simulink library "NeuroMuscularLibrary"  (R2014b)
settings: Solver=ode45  StartTime=0.0  StopTime=10.0  RelTol=1e-3
values from neighbouring files (symbols this model uses):
  c = 0.05    [BodyMechParams.m]
  c_jointstop = 0.3 / (pi/180)    (= 17.1887338539)    [BodyMechParams.m]
  DeltaThRef = 2e-3    (= 0.002)    [BodyMechParams.m]
  eref = 0.04    [BodyMechParams.m]
  footBallToAnkleDist = 0.16    [BodyMechParams.m]
  footBallToCenterDist = footLength/2    (= 0.1)    [BodyMechParams.m]
  footBallToHeelDist = footLength    (= 0.2)    [BodyMechParams.m]
  footCenterToCGDist = 0.14 - footBallToCenterDist    (= 0.04)    [BodyMechParams.m]
  footInertia = 0.005    [BodyMechParams.m]
  footLength = 0.2    [BodyMechParams.m]
  footMass = 1.25    [BodyMechParams.m]
  g = 9.80665    [BodyMechParams.m]
  groundTheta = [atan(diff(groundZ)./diff(groundX)), 0]    [generateGround.m]
  groundZ = groundZ * stepSize/(largestStep+eps)    [generateGround.m]
  hatHipToCenterDistLen = hatLength/2    (= 0.4)    [BodyMechParams.m]
  hatInertia = 3    [BodyMechParams.m]
  hatLeftHipToCenterDistWidth = .15    (= 0.15)    [BodyMechParams.m]
  hatLength = 0.8    [BodyMechParams.m]
  hatMass = 53.5    [BodyMechParams.m]
  hatThickness = 0.2    [BodyMechParams.m]
  hatWidth = 0.4    [BodyMechParams.m]
  K = 5    [BodyMechParams.m]
  k_gn = k_gz    (= 78453.2)    [BodyMechParams.m]
  k_gt = k_gz    (= 78453.2)    [BodyMechParams.m]
  k_pressure = hatMass * g / DeltaThRef    (= 262327.8875)    [BodyMechParams.m]
  loptGAS = 0.05    [BodyMechParams.m]
  loptGLU = 0.11    [BodyMechParams.m]
  loptHAM = 0.10    (= 0.1)    [BodyMechParams.m]
  loptHFL = 0.11    [BodyMechParams.m]
  loptSOL = 0.04    [BodyMechParams.m]
  loptTA = 0.06    [BodyMechParams.m]
  loptVAS = 0.08    [BodyMechParams.m]
  lslackGAS = 0.40    (= 0.4)    [BodyMechParams.m]
  lslackGLU = 0.13    [BodyMechParams.m]
  lslackHAM = 0.31    [BodyMechParams.m]
  lslackHFL = 0.10    (= 0.1)    [BodyMechParams.m]
  lslackSOL = 0.26    [BodyMechParams.m]
  lslackTA = 0.24    [BodyMechParams.m]
  lslackVAS = 0.23    [BodyMechParams.m]
  mu_slide = 0.8    [BodyMechParams.m]
  mu_stick = 0.9    [BodyMechParams.m]
  N = 1.5    [BodyMechParams.m]    (also in cmaes.m = size(x,1))
  phimaxGASa = 20*pi/180    (= 0.349065850399)    [BodyMechParams.m]
  phimaxGASk = 40*pi/180    (= 0.698131700798)    [BodyMechParams.m]
  phimaxHAMk = 0*pi/180    (= 0)    [BodyMechParams.m]
  phimaxSOL = 20*pi/180    (= 0.349065850399)    [BodyMechParams.m]
  phimaxTA = -10*pi/180    (= -0.174532925199)    [BodyMechParams.m]
  phimaxVAS = 15*pi/180    (= 0.261799387799)    [BodyMechParams.m]
  phirefGASa = -10*pi/180    (= -0.174532925199)    [BodyMechParams.m]
  phirefGASk = 15*pi/180    (= 0.261799387799)    [BodyMechParams.m]
  phirefGLU = -30*pi/180    (= -0.523598775598)    [BodyMechParams.m]
  phirefHAMh = -25*pi/180    (= -0.436332312999)    [BodyMechParams.m]
  phirefHAMk = 0*pi/180    (= 0)    [BodyMechParams.m]
  phirefHFL = 0*pi/180    (= 0)    [BodyMechParams.m]
  phirefSOL = -10*pi/180    (= -0.174532925199)    [BodyMechParams.m]
  phirefTA = 20*pi/180    (= 0.349065850399)    [BodyMechParams.m]
  phirefVAS = 55*pi/180    (= 0.959931088597)    [BodyMechParams.m]
  rGASa = 0.05    [BodyMechParams.m]
  rGASk = 0.05    [BodyMechParams.m]
  rGLU = 0.10    (= 0.1)    [BodyMechParams.m]
  rHAMh = 0.08    [BodyMechParams.m]
  rHAMk = 0.05    [BodyMechParams.m]
  rHFL = 0.10    (= 0.1)    [BodyMechParams.m]
  rhoGASa = 0.7    [BodyMechParams.m]
  rhoGASk = 0.7    [BodyMechParams.m]
  rhoGLU = 0.5    [BodyMechParams.m]
  rhoHAMh = 0.7    [BodyMechParams.m]
  rhoHAMk = 0.7    [BodyMechParams.m]
  rhoHFL = 0.5    [BodyMechParams.m]
  rhoSOL = 0.5    [BodyMechParams.m]
  rhoTA = 0.7    [BodyMechParams.m]
  rhoVAS = 0.7    [BodyMechParams.m]
  rSOL = 0.05    [BodyMechParams.m]
  rTA = 0.04    [BodyMechParams.m]
  rVAS = 0.06    [BodyMechParams.m]
  s = x(1:N-1,:).^2 + x(2:N,:).^2    [cmaes.m]
  shankAnkleToCenterDist = shankLength/2    (= 0.25)    [BodyMechParams.m]
  shankAnkleToKneeDist = shankLength    (= 0.5)    [BodyMechParams.m]
  shankCenterToCGDist = 0.3 - shankAnkleToCenterDist    (= 0.05)    [BodyMechParams.m]
  shankInertia = 0.05    [BodyMechParams.m]
  shankLength = 0.5    [BodyMechParams.m]
  shankMass = 3.5    [BodyMechParams.m]
  tau = 0.01    [BodyMechParams.m]
  thighCenterToCGDist = 0.3 - thighKneeToCenterDist    (= 0.05)    [BodyMechParams.m]
  thighInertia = 0.15    [BodyMechParams.m]
  thighKneeToCenterDist = thighLength/2    (= 0.25)    [BodyMechParams.m]
  thighKneeToHipDist = thighLength    (= 0.5)    [BodyMechParams.m]
  thighLength = 0.5    [BodyMechParams.m]
  thighMass = 8.5    [BodyMechParams.m]
  v_gn_max = v_gz_max    (= 0.03)    [BodyMechParams.m]
  v_gt_max = v_gz_max    (= 0.03)    [BodyMechParams.m]
  v_max_pressure = 0.5    [BodyMechParams.m]
  vLimit = 0.01    [BodyMechParams.m]
  w = 0.56    [BodyMechParams.m]    (also in cmaes.m = ones(size(x,1)))
  w_max_jointstop = 1 * pi/180    (= 0.0174532925199)    [BodyMechParams.m]
undefined symbols (not defined in the file or in its folder): ankleBackDriveGain, ankleDgain, ankleFilterPID, ankleFilterSEA, ankleGearEff, ankleGearRatio, ankleIgain, ankleInitialAngle, ankleInputMass, ankleParallelSpringDamping, ankleParallelSpringOffset, ankleParallelSpringStiffness, anklePgain, ankleSEADamping, ankleSEAStiffness, ankleTendonMass, deltaLegAngleThr, footMassp, FourBarL1, FourBarL3, GainGAS, GainGLU, GainHAM, GainKneeOverExt, GainSOL, GainSOLTA, GainTA, GainVAS, hipDGain, hipPGain, Kglu, kneeAngleOffset, kneeBackDriveGain, kneeDgain, kneeExtendGain, kneeFilterPID, kneeFilterSEA, kneeFlexGain, kneeGearEff, kneeGearRatio, kneeHoldGain1, kneeHoldGain2, kneeIgain, kneeInitialAngle, kneePgain, kneeSEADamping, kneeSEAStiffness, kneeStatorMass, kneeStopGain, legAngleFilter, legAngleSpeedMax, legLengthClr, motorBackEMF, motorInductance, motorMaxCurrent, motorMaxVoltage, motorResistance, motorRotorInertia, motorRotorMass, motorTorsionalConst ... (+19)
undefined symbols (not defined in the file): ankleCJointstop, ankleIntCoulomb, ankleIntDamping, ankleIntStatic, anklePlantarLimit, ankleWMaxJointstop, dryFrictionDamping, dryFrictionStiffness, dryFrictionVelThresh, FmaxGLU, FT_GLU, kneeCJointstop, kneeExtCoulomb, kneeExtDamping, kneeExtStatic, kneeIntCoulomb, kneeIntDamping, kneeIntStatic, kneeWMaxJointstop, phiKneeUpLimit, RGainGAS, RGainGLU, RGainHAM, RGainHAMCut, RGainKneeOverExt, RGainSOL, RGainSOLTA, RGainTA, RGainVAS, RhipDGain, RhipPGain, RKglu, RkneeExtendGain, RkneeFlexGain, RkneeHoldGain1, RkneeHoldGain2, RkneeStopGain, RlegAngleFilter, RlegLengthClr, RPosGainGG, RSpeedGainGG
libraries: sm_lib x90, nesl_utility x44, simulink x18, dspswit3 x10, NeuroMuscularLibrary x8, simulink_extras x2
(part 2 of 5)

== system NeuroMuscularLibrary/Leg Angle//Length ==
  Constant : Constant  Value=pi
  Demux : Demux  Outputs=2
  Mux : Mux  Inputs=3
  Mux1 : Mux  Inputs=3
  PS-Simulink Converter{,1..6} (7 alike) : nesl_utility/PS-Simulink Converter  PhysicalDomain=network_engine_domain  SubClassName=ps_output  LeftPortType=input  RightPortType=output  PseudoPeriodic=off  Frequencies=[]  Unit=m  AffineConversion=off
  Position Sensor : sm_lib/Frames and Transforms/Transform Sensor  MeasurementFrame=World  SenseAngle=off  SenseAxis=off  SenseAngle1=off  SenseAngle2=off  SenseAngle3=off  SenseQ=off  SenseR=off  SenseOmegaX=off  SenseOmegaY=off  SenseOmegaZ=off  SenseOmega1=off  SenseOmega2=off  SenseOmega3=off  SenseQDot=off  SenseRDot=off  SenseAlphaX=off  SenseAlphaY=off  SenseAlphaZ=off  SenseAlpha1=off  SenseAlpha2=off  SenseAlpha3=off  SenseQDDot=off  SenseRDDot=off  SenseX=on  SenseY=on  SenseZ=on  SenseRad=off  SenseAzim=off  SenseDist=off  SenseInc=off  SenseXDot=off  SenseYDot=off  SenseZDot=off  SenseRadDot=off  SenseAzimDot=off  SenseDistDot=off  SenseIncDot=off  SenseXDDot=off  SenseYDDot=off  SenseZDDot=off  SenseRadDDot=off  SenseAzimDDot=off  SenseDistDDot=off  SenseIncDDot=off  BlockFunction=simmechanics.library.frames_transforms.transform_sensor
  Position Sensor1 : sm_lib/Frames and Transforms/Transform Sensor  MeasurementFrame=World  SenseAngle=off  SenseAxis=off  SenseAngle1=off  SenseAngle2=off  SenseAngle3=off  SenseQ=off  SenseR=off  SenseOmegaX=off  SenseOmegaY=off  SenseOmegaZ=off  SenseOmega1=off  SenseOmega2=off  SenseOmega3=off  SenseQDot=off  SenseRDot=off  SenseAlphaX=off  SenseAlphaY=off  SenseAlphaZ=off  SenseAlpha1=off  SenseAlpha2=off  SenseAlpha3=off  SenseQDDot=off  SenseRDDot=off  SenseX=on  SenseY=on  SenseZ=on  SenseRad=off  SenseAzim=off  SenseDist=off  SenseInc=off  SenseXDot=off  SenseYDot=off  SenseZDot=off  SenseRadDot=off  SenseAzimDot=off  SenseDistDot=off  SenseIncDot=off  SenseXDDot=off  SenseYDDot=off  SenseZDDot=off  SenseRadDDot=off  SenseAzimDDot=off  SenseDistDDot=off  SenseIncDDot=off  BlockFunction=simmechanics.library.frames_transforms.transform_sensor
  Selector : Selector  InputPortWidth=3  Indices=[3 1]
  Subtract : Sum  Inputs=+-
  Sum : Sum  Inputs=|-+
  Transform Sensor : sm_lib/Frames and Transforms/Transform Sensor  MeasurementFrame=World  SenseAngle=off  SenseAxis=off  SenseAngle1=off  SenseAngle2=off  SenseAngle3=off  SenseQ=off  SenseR=off  SenseOmegaX=off  SenseOmegaY=off  SenseOmegaZ=off  SenseOmega1=off  SenseOmega2=off  SenseOmega3=off  SenseQDot=off  SenseRDot=off  SenseAlphaX=off  SenseAlphaY=off  SenseAlphaZ=off  SenseAlpha1=off  SenseAlpha2=off  SenseAlpha3=off  SenseQDDot=off  SenseRDDot=off  SenseX=off  SenseY=off  SenseZ=off  SenseRad=off  SenseAzim=off  SenseDist=on  SenseInc=off  SenseXDot=off  SenseYDot=off  SenseZDot=off  SenseRadDot=off  SenseAzimDot=off  SenseDistDot=off  SenseIncDot=off  SenseXDDot=off  SenseYDDot=off  SenseZDDot=off  SenseRadDDot=off  SenseAzimDDot=off  SenseDistDDot=off  SenseIncDDot=off  BlockFunction=simmechanics.library.frames_transforms.transform_sensor
  Trigonometric Function : Trigonometry  Operator=atan2  OutputSignalType=real
  World Frame : sm_lib/Frames and Transforms/World Frame  BlockFunction=simmechanics.library.frames_transforms.world_frame
  Hip : PMIOPort  Port=1  Side=Left
  Ankle : PMIOPort  Port=2  Side=Left
  Leg Angle : Outport
  Leg Length : Outport  Port=2
  wires:
  PS-Simulink Converter6/1 -> Leg Length/1
  PS-Simulink Converter2/1 -> Mux/3
  PS-Simulink Converter/1 -> Mux/1
  PS-Simulink Converter1/1 -> Mux/2
  PS-Simulink Converter5/1 -> Mux1/3
  PS-Simulink Converter3/1 -> Mux1/1
  PS-Simulink Converter4/1 -> Mux1/2
  Mux/1 -> Subtract/1
  Mux1/1 -> Subtract/2
  Trigonometric Function/1 -> Sum/1
  Sum/1 -> Leg Angle/1
  Constant/1 -> Sum/2
  Subtract/1 -> Selector/1
  Selector/1 -> Demux/1
  Demux/1 -> Trigonometric Function/1
  Demux/2 -> Trigonometric Function/2
  connections:
  PS-Simulink Converter6/LConn1 -- Transform Sensor/RConn2
  PS-Simulink Converter2/LConn1 -- Position Sensor/RConn4
  PS-Simulink Converter/LConn1 -- Position Sensor/RConn2
  Transform Sensor/RConn1 -- Hip/RConn1 -- Position Sensor/RConn1
  PS-Simulink Converter1/LConn1 -- Position Sensor/RConn3
  World Frame/RConn1 -- Position Sensor/LConn1 -- Position Sensor1/LConn1
  PS-Simulink Converter4/LConn1 -- Position Sensor1/RConn3
  PS-Simulink Converter5/LConn1 -- Position Sensor1/RConn4
  PS-Simulink Converter3/LConn1 -- Position Sensor1/RConn2
  Transform Sensor/LConn1 -- Ankle/RConn1 -- Position Sensor1/RConn1

== system NeuroMuscularLibrary/Lower Thigh ==
  Knee Solid : sm_lib/Body Elements/Solid  InertiaType=Custom  Mass=thighMass*ThPos  MassUnits=kg  CenterOfMass=[0 0 thighCenterToCGDist*ThPos]  CenterOfMassUnits=m  MomentsOfInertia=[thighInertia*(ThPos)^3 0 0]  MomentsOfInertiaUnits=kg*m^2  ProductsOfInertia=[0 0 0]  ProductsOfInertiaUnits=kg*m^2  DensityBased=on  Density=1000  DensityUnits=kg/(m^3)  GraphicType=FromGeometry  MarkerShape=Sphere  MarkerSize=10  MarkerSizeUnits=m  GraphicVisPropType=SimpleVisualProperties  GraphicDiffuseColor=[0.5 0.5 0.5]  GraphicSpecularColor=[0.5 0.5 0.5 1.0]  GraphicAmbientColor=[0.15 0.15 0.15 1.0]  GraphicEmissiveColor=[0.0 0.0 0.0 1.0]  GraphicShininess=75  GraphicOpacity=1.0  GeometryShape=Cylinder  RectangleSize=[1 1]  RectangleSizeUnits=m  BrickDimensions=[1.05 .1]  BrickDimensionUnits=m  CylinderRadius=.075  CylinderRadiusUnits=m  CylinderLength=thighLength*ThPos  CylinderLengthUnits=m  SphereRadius=1  SphereRadiusUnits=m  EllipsoidRadii=[1 1 1]  EllipsoidRadiiUnits=m  ExtrusionCrossSection=[1 1; -1 1; -1 -1; 1 -1]  ExtrusionCrossSectionUnits=m  ExtrusionLength=1  ExtrusionLengthUnits=m  PolygonNumSides=3  PolygonOuterRadius=1  PolygonOuterRadiusUnits=m  ExtGeomFileType=STL  ExtGeomFileUnits=m  RevolutionCrossSection=[1 1; 1 -1; 2 -1; 2 1]  RevolutionCrossSectionUnits=m  RevolutionExtent=Full  RevolutionAngle=180  RevolutionAngleUnits=deg  BlockFunction=simmechanics.library.body_elements.solid
  Knee to Center : sm_lib/Frames and Transforms/Rigid Transform  TranslationMethod=Cartesian  TranslationLengthUnit=m  TranslationStandardAxis=+Z  TranslationStandardOffset=0  TranslationCartesianOffset=[0 thighKneeToCenterDist*ThPos 0]  TranslationROffset=0  TranslationROffsetUnits=m  TranslationZOffset=0  TranslationZOffsetUnits=m  TranslationThetaOffset=0  TranslationThetaOffsetUnits=deg  RotationMethod=AlignedAxes  RotationAngleUnits=deg  RotationStandardAxis=+Z  RotationAngle=0  RotationArbitraryAxis=[0 0 1]  FollAlignAxisA=+Z  BaseAlignAxisA=+Y  FollAlignAxisB=+X  BaseAlignAxisB=+X  RotationMatrix=[1 0 0; 0 1 0; 0 0 1]  BlockFunction=simmechanics.library.frames_transforms.rigid_transform
  Knee to Sensor Sheet : sm_lib/Frames and Transforms/Rigid Transform  TranslationMethod=Cartesian  TranslationLengthUnit=m  TranslationStandardAxis=+Z  TranslationStandardOffset=0  TranslationCartesianOffset=[0 thighKneeToHipDist*ThPos 0]  TranslationROffset=0  TranslationROffsetUnits=m  TranslationZOffset=0  TranslationZOffsetUnits=m  TranslationThetaOffset=0  TranslationThetaOffsetUnits=deg  RotationMethod=None  RotationAngleUnits=deg  RotationStandardAxis=+Z  RotationAngle=0  RotationArbitraryAxis=[0 0 1]  FollAlignAxisA=+Z  BaseAlignAxisA=+X  FollAlignAxisB=+Y  BaseAlignAxisB=+Y  RotationMatrix=[1 0 0; 0 1 0; 0 0 1]  BlockFunction=simmechanics.library.frames_transforms.rigid_transform
  Thigh CG : sm_lib/Frames and Transforms/Reference Frame  BlockFunction=simmechanics.library.frames_transforms.reference_frame
  Thigh Center to CG : sm_lib/Frames and Transforms/Rigid Transform  TranslationMethod=Cartesian  TranslationLengthUnit=m  TranslationStandardAxis=+Z  TranslationStandardOffset=0  TranslationCartesianOffset=[0 0 thighCenterToCGDist*ThPos]  TranslationROffset=0  TranslationROffsetUnits=m  TranslationZOffset=0  TranslationZOffsetUnits=m  TranslationThetaOffset=0  TranslationThetaOffsetUnits=deg  RotationMethod=None  RotationAngleUnits=deg  RotationStandardAxis=+Z  RotationAngle=0  RotationArbitraryAxis=[0 0 1]  FollAlignAxisA=+X  BaseAlignAxisA=+Y  FollAlignAxisB=+Y  BaseAlignAxisB=+Z  RotationMatrix=[1 0 0; 0 1 0; 0 0 1]  BlockFunction=simmechanics.library.frames_transforms.rigid_transform
  Knee : PMIOPort  Port=1  Side=Left
  Sensor Sheet : PMIOPort  Port=2  Side=Right
  connections:
  Knee/RConn1 -- Knee to Center/LConn1 -- Knee to Sensor Sheet/LConn1
  Knee to Center/RConn1 -- Knee Solid/RConn1 -- Thigh Center to CG/LConn1
  Knee to Sensor Sheet/RConn1 -- Sensor Sheet/RConn1
  Thigh Center to CG/RConn1 -- Thigh CG/RConn1

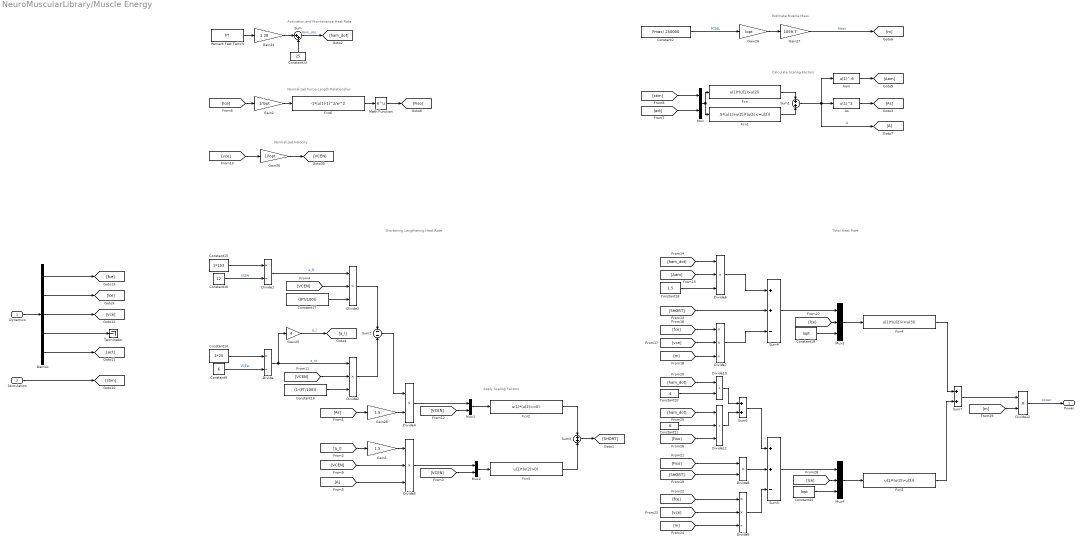
== system NeuroMuscularLibrary/Muscle Energy ==
  note: Total Heat Rate
  note: Estimate Muscle Mass
  note: Calculate Scaling Factors
  note: Apply Scaling Factors
  note: Shortening Lengthening Heat Rate
  note: Normalized Velocity
  note: Normalized Force-Length Relationship
  note: Activation and Maintenance Heat Rate
  Dynamics : Inport
  Stimulation : Inport  Port=2
  "Aam " : Fcn  Expr=u(1)^.6
  As : Fcn  Expr=u(1)^2
  Constant10 : Constant  Value=12
  Constant13 : Constant  Value=25
  Constant14 : Constant  Value=4*25
  Constant15 : Constant  Value=1*153
  Constant16 : Constant  Value=(1-(FT/100))
  Constant17 : Constant  Value=((FT/100))
  Constant18 : Constant  Value=1.5
  Constant19 : Constant  Value=lopt
  Constant2 : Constant  Value=Fmax/ 250000
  Constant20 : Constant  Value=.4
  Constant21 : Constant  Value=.6
  Constant22 : Constant  Value=lopt
  Constant9 : Constant  Value=6
  Demux : Demux  Outputs=5
  Divide : Product  Inputs=*/
  Divide1 : Product  Inputs=*/
  Divide{4,8,10,12} (4 alike) : Product  Inputs=**
  Divide{2..3,5..6,11} (5 alike) : Product  Inputs=***
  Divide7 : Product  Inputs=**/
  Divide9 : Product  Inputs=**/
  Fcn : Fcn  Expr=u(1)*(u(1)>u(2))
  Fcn1 : Fcn  Expr=.5*(u(1)+u(2))*(u(1)<=u(2))
  Fcn2 : Fcn  Expr=u(1)*(u(2)<=0)
  Fcn3 : Fcn  Expr=u(1)*(u(2)>0)
  Fcn4 : Fcn  Expr=u(1)*(u(2)<=u(3))
  Fcn5 : Fcn  Expr=u(1)*(u(2)>u(3))
  Fcn6 : Fcn  Expr=-1*(u(1)-1)^2/w^2
  Gain1 : Gain  Gain=1.5
  Gain2 : Gain  Gain=1/lopt
  Gain24 : Gain  Gain=1.28
  Gain25 : Gain  Gain=4
  Gain26 : Gain  Gain=lopt
  Gain27 : Gain  Gain=1059.7
  Gain28 : Gain  Gain=1.5
  Gain30 : Gain  Gain=1/lopt
  Math Function : Math  SaturateOnIntegerOverflow=on
  Mux : Mux  Inputs=2
  Mux1 : Mux  Inputs=2
  Mux2 : Mux  Inputs=2
  Mux3 : Mux  Inputs=3
  Mux4 : Mux  Inputs=3
  Percent Fast Twitch : Constant  Value=FT
  Sum : Sum  Inputs=|++
  Sum1 : Sum  Inputs=+|+
  Sum2 : Sum  Inputs=-|-
  Sum3 : Sum  Inputs=+|+
  Sum4 : Sum  Inputs=++-
  Sum5 : Sum  Inputs=++-
  Sum6 : Sum
  Sum7 : Sum
  Terminator : Terminator
  Power : Outport
  wires:
  Gain2/1 -> Fcn6/1
  [lce] -> Gain2/1
  Demux/4 -> Terminator/1
  Demux/5 -> [act]
  Demux/3 -> [vce]
  Demux/2 -> [lce]
  Demux/1 -> [fce]
  Stimulation/1 -> [stim]
  Dynamics/1 -> Demux/1
  [As] -> Gain28/1
  Fcn2/1 -> Sum3/1
  Sum3/1 -> [SHORT]
  Mux2/1 -> Fcn3/1
  Gain30/1 -> [VCEN]
  Gain27/1 -> [m]  "Mass"
  Constant9/1 -> Divide/2  "VCEst"
  Gain28/1 -> Divide4/2
  [lce] -> Mux3/2
  Mux3/1 -> Fcn4/1
  [SHORT] -> Divide8/2
  Constant2/1 -> Gain26/1  "PCSAL"
  Constant21/1 -> Divide11/2
  [VCEN] -> Mux2/2
  Percent Fast Twitch/1 -> Gain24/1
  Mux/1 -> Fcn/1, Fcn1/1
  Sum/1 -> [ham_dot]  "Ham_dot"
  [fce] -> Divide9/1
  [m] -> Divide7/3
  Sum2/1 -> Divide4/1
  Constant20/1 -> Divide10/2
  As/1 -> [As]
  Divide8/1 -> Sum5/2
  Constant13/1 -> Sum/2
  Divide7/1 -> Sum4/3
  [vce] -> Divide9/2
  Fcn/1 -> Sum1/1
  Fcn1/1 -> Sum1/2
  [VCEN] -> Divide3/2
  Mux1/1 -> Fcn2/1
  Divide4/1 -> Mux1/1
  Constant15/1 -> Divide1/1
  Constant18/1 -> Divide6/3
  Sum1/1 -> [A], As/1, "Aam "/1  "A"
  [ham_dot] -> Divide6/1
  Divide/1 -> Divide2/1, Gain25/1  "a_st"
  Divide6/1 -> Sum4/1
  Constant14/1 -> Divide/1
  Divide5/1 -> Mux2/1
  Constant22/1 -> Mux4/3
  Fcn3/1 -> Sum3/2
  Sum7/1 -> Divide12/1
  [VCEN] -> Mux1/2
  Divide1/1 -> Divide3/1  "a_ft"
  [VCEN] -> Divide2/2
  Divide2/1 -> Sum2/2
  Constant10/1 -> Divide1/2  "VCEft"
  "Aam "/1 -> [Aam]
  Math Function/1 -> [Fiso]
  Gain25/1 -> [a_l]  "a_l"
  Divide3/1 -> Sum2/1
  [vce] -> Divide7/2
  [Fiso] -> Divide11/3
  Constant17/1 -> Divide3/3
  Constant16/1 -> Divide2/3
  Gain1/1 -> Divide5/1
  [Aam] -> Divide6/2
  [a_l] -> Gain1/1
  [VCEN] -> Divide5/2
  Fcn5/1 -> Sum7/2
  Mux4/1 -> Fcn5/1
  Constant19/1 -> Mux3/3
  [SHORT] -> Sum4/2
  Sum6/1 -> Sum5/1
  Sum5/1 -> Mux4/1
  [ham_dot] -> Divide10/1
  [lce] -> Mux4/2
  [m] -> Divide9/3
  Divide11/1 -> Sum6/2
  [ham_dot] -> Divide11/1
  [A] -> Divide5/3
  Fcn6/1 -> Math Function/1
  [Fiso] -> Divide8/1
  Fcn4/1 -> Sum7/1
  Divide12/1 -> Power/1  "power"
  Sum4/1 -> Mux3/1
  Divide9/1 -> Sum5/3
  Divide10/1 -> Sum6/1
  Gain24/1 -> Sum/1
  Gain26/1 -> Gain27/1
  [stim] -> Mux/1
  [act] -> Mux/2
  [vce] -> Gain30/1
  [fce] -> Divide7/1
  [m] -> Divide12/2

== system NeuroMuscularLibrary/Overextension Joint Limit ==
  note: Knee/Hip Joint Limits
  phi [rad] : Inport
  dphi [rad/s] : Inport  Port=2
  Gain1 : Gain  Gain=ext
  Gain2 : Gain  Gain=-ext
  Gain3 : Gain  Gain=c_jointstop
  Gain4 : Gain  Gain=1/w_max_jointstop
  Gain5 : Gain  Gain=ext
  Limit Ankle Range : simulink/Logic and Bit Operations/Interval Test  Commented=on  IntervalClosedRight=on  uplimit=185*pi/180  IntervalClosedLeft=on  lowlimit=40*pi/180  OutDataTypeStr=boolean
  Logical Operator3 : Logic  Commented=on  Operator=NOT  AllPortsSameDT=off  OutDataTypeStr=boolean
  Mux3 : Mux  Inputs=2
  Overextension Torque : Fcn  Expr="- u(1)  *  (1-u(2)) * (u(2)<1) * (u(1)>0)"
  Stop Simulation1 : Stop  Commented=on
  Sum : Sum  Inputs=|+-
  overextension angle : Constant  Value=phiUpLimit
  M_stop [Nm] : Outport
  wires:
  Gain5/1 -> M_stop [Nm]/1
  Overextension Torque/1 -> Gain5/1
  Logical Operator3/1 -> Stop Simulation1/1
  Limit Ankle Range/1 -> Logical Operator3/1
  Gain2/1 -> Mux3/2
  Gain4/1 -> Gain2/1
  Sum/1 -> Gain3/1
  phi [rad]/1 -> Limit Ankle Range/1, Sum/1
  overextension angle/1 -> Sum/2
  dphi [rad/s]/1 -> Gain4/1
  Mux3/1 -> Overextension Torque/1
  Gain3/1 -> Gain1/1
  Gain1/1 -> Mux3/1

== system NeuroMuscularLibrary/Overextension//Overflexion Joint Limit ==
  note: Overextension/Overflexion Joint Limit
  phi [rad] : Inport
  dphi [rad/s] : Inport  Port=2
  Gain1 : Gain  Gain=c_jointstop
  Gain2 : Gain  Gain=-1
  Gain3 : Gain  Gain=c_jointstop
  Gain4 : Gain  Gain=1/w_max_jointstop
  Limit Range : simulink/Logic and Bit Operations/Interval Test  Commented=on  IntervalClosedRight=on  uplimit=phi12_UpLimit + 40*pi/180  IntervalClosedLeft=on  lowlimit=phi12_LowLimit - 40*pi/180  OutDataTypeStr=boolean
  Logical Operator3 : Logic  Commented=on  Operator=NOT  AllPortsSameDT=off  OutDataTypeStr=boolean
  Mux1 : Mux  Inputs=2
  Mux3 : Mux  Inputs=2
  Overextension Torque : Fcn  Expr="- u(1)  *  (1-u(2)) * (u(2)<1) * (u(1)>0)"
  Overflexion Torque : Fcn  Expr="- u(1)  *  (1-u(2)) * (u(2)<1) * (u(1)<0)"
  Stop Simulation1 : Stop  Commented=on
  Sum : Sum  Inputs=|+-
  Sum1 : Sum  Inputs=|+-
  Sum2 : Sum
  overextension angle : Constant  Value=phiUpLimit
  overflexion angle : Constant  Value=phiLowLimit
  M_stop [Nm] : Outport
  wires:
  Mux3/1 -> Overextension Torque/1
  Gain3/1 -> Mux3/1
  dphi [rad/s]/1 -> Gain4/1
  overextension angle/1 -> Sum/2
  phi [rad]/1 -> Sum/1, Sum1/1, Limit Range/1
  Sum/1 -> Gain3/1
  Gain4/1 -> Gain2/1, Mux1/2
  Gain1/1 -> Mux1/1
  Sum1/1 -> Gain1/1
  overflexion angle/1 -> Sum1/2
  Mux1/1 -> Overflexion Torque/1
  Sum2/1 -> M_stop [Nm]/1
  Gain2/1 -> Mux3/2
  Overflexion Torque/1 -> Sum2/2
  Overextension Torque/1 -> Sum2/1
  Limit Range/1 -> Logical Operator3/1
  Logical Operator3/1 -> Stop Simulation1/1

== system NeuroMuscularLibrary/Pos//Rot Sensor ==
  Gain2 : Gain  Gain=-1
  Mux : Mux  Inputs=3
  PS-Simulink Converter : nesl_utility/PS-Simulink Converter  PhysicalDomain=network_engine_domain  SubClassName=ps_output  LeftPortType=input  RightPortType=output  PseudoPeriodic=off  Frequencies=[]  Unit=m  AffineConversion=off
  PS-Simulink Converter1 : nesl_utility/PS-Simulink Converter  PhysicalDomain=network_engine_domain  SubClassName=ps_output  LeftPortType=input  RightPortType=output  PseudoPeriodic=off  Frequencies=[]  Unit=m  AffineConversion=off
  PS-Simulink Converter2 : nesl_utility/PS-Simulink Converter  PhysicalDomain=network_engine_domain  SubClassName=ps_output  LeftPortType=input  RightPortType=output  PseudoPeriodic=off  Frequencies=[]  Unit=m  AffineConversion=off
  PS-Simulink Converter3 : nesl_utility/PS-Simulink Converter  PhysicalDomain=network_engine_domain  SubClassName=ps_output  LeftPortType=input  RightPortType=output  PseudoPeriodic=off  Frequencies=[]  Unit=rad  AffineConversion=off
  PS-Simulink Converter4 : nesl_utility/PS-Simulink Converter  PhysicalDomain=network_engine_domain  SubClassName=ps_output  LeftPortType=input  RightPortType=output  PseudoPeriodic=off  Frequencies=[]  Unit=rad  AffineConversion=off
  Position Sensor : sm_lib/Frames and Transforms/Transform Sensor  MeasurementFrame=World  SenseAngle=on  SenseAxis=on  SenseAngle1=off  SenseAngle2=off  SenseAngle3=off  SenseQ=off  SenseR=off  SenseOmegaX=off  SenseOmegaY=off  SenseOmegaZ=off  SenseOmega1=off  SenseOmega2=off  SenseOmega3=off  SenseQDot=off  SenseRDot=off  SenseAlphaX=off  SenseAlphaY=off  SenseAlphaZ=off  SenseAlpha1=off  SenseAlpha2=off  SenseAlpha3=off  SenseQDDot=off  SenseRDDot=off  SenseX=on  SenseY=on  SenseZ=on  SenseRad=off  SenseAzim=off  SenseDist=off  SenseInc=off  SenseXDot=off  SenseYDot=off  SenseZDot=off  SenseRadDot=off  SenseAzimDot=off  SenseDistDot=off  SenseIncDot=off  SenseXDDot=off  SenseYDDot=off  SenseZDDot=off  SenseRadDDot=off  SenseAzimDDot=off  SenseDistDDot=off  SenseIncDDot=off  BlockFunction=simmechanics.library.frames_transforms.transform_sensor
  Product : Product
  Selector : Selector  InputPortWidth=3  Indices=[3]
  Sign : Signum
  F : PMIOPort  Port=1  Side=Left
  B : PMIOPort  Port=2  Side=Right
  Position : Outport
  Rotation : Outport  Port=2
  wires:
  PS-Simulink Converter1/1 -> Mux/2
  PS-Simulink Converter/1 -> Mux/1
  Mux/1 -> Position/1
  PS-Simulink Converter2/1 -> Mux/3
  PS-Simulink Converter4/1 -> Selector/1
  Selector/1 -> Sign/1
  PS-Simulink Converter3/1 -> Product/1
  Sign/1 -> Product/2
  Gain2/1 -> Rotation/1
  Product/1 -> Gain2/1
  connections:
  Position Sensor/RConn1 -- F/RConn1
  PS-Simulink Converter3/LConn1 -- Position Sensor/RConn2
  B/RConn1 -- Position Sensor/LConn1
  Position Sensor/RConn4 -- PS-Simulink Converter/LConn1
  PS-Simulink Converter1/LConn1 -- Position Sensor/RConn5
  PS-Simulink Converter2/LConn1 -- Position Sensor/RConn6
  PS-Simulink Converter4/LConn1 -- Position Sensor/RConn3

== system NeuroMuscularLibrary/Position Sensor ==
  Mux : Mux  Inputs=3
  PS-Simulink Converter : nesl_utility/PS-Simulink Converter  PhysicalDomain=network_engine_domain  SubClassName=ps_output  LeftPortType=input  RightPortType=output  PseudoPeriodic=off  Frequencies=[]  Unit=m  AffineConversion=off
  PS-Simulink Converter1 : nesl_utility/PS-Simulink Converter  PhysicalDomain=network_engine_domain  SubClassName=ps_output  LeftPortType=input  RightPortType=output  PseudoPeriodic=off  Frequencies=[]  Unit=m  AffineConversion=off
  PS-Simulink Converter2 : nesl_utility/PS-Simulink Converter  PhysicalDomain=network_engine_domain  SubClassName=ps_output  LeftPortType=input  RightPortType=output  PseudoPeriodic=off  Frequencies=[]  Unit=m  AffineConversion=off
  Position Sensor : sm_lib/Frames and Transforms/Transform Sensor  MeasurementFrame=World  SenseAngle=off  SenseAxis=off  SenseAngle1=off  SenseAngle2=off  SenseAngle3=off  SenseQ=off  SenseR=off  SenseOmegaX=off  SenseOmegaY=off  SenseOmegaZ=off  SenseOmega1=off  SenseOmega2=off  SenseOmega3=off  SenseQDot=off  SenseRDot=off  SenseAlphaX=off  SenseAlphaY=off  SenseAlphaZ=off  SenseAlpha1=off  SenseAlpha2=off  SenseAlpha3=off  SenseQDDot=off  SenseRDDot=off  SenseX=on  SenseY=on  SenseZ=on  SenseRad=off  SenseAzim=off  SenseDist=off  SenseInc=off  SenseXDot=off  SenseYDot=off  SenseZDot=off  SenseRadDot=off  SenseAzimDot=off  SenseDistDot=off  SenseIncDot=off  SenseXDDot=off  SenseYDDot=off  SenseZDDot=off  SenseRadDDot=off  SenseAzimDDot=off  SenseDistDDot=off  SenseIncDDot=off  BlockFunction=simmechanics.library.frames_transforms.transform_sensor
  World Frame : sm_lib/Frames and Transforms/World Frame  BlockFunction=simmechanics.library.frames_transforms.world_frame
  Frame : PMIOPort  Port=1  Side=Left
  Position : Outport
  wires:
  PS-Simulink Converter2/1 -> Mux/3
  Mux/1 -> Position/1
  PS-Simulink Converter/1 -> Mux/1
  PS-Simulink Converter1/1 -> Mux/2
  connections:
  PS-Simulink Converter2/LConn1 -- Position Sensor/RConn4
  PS-Simulink Converter/LConn1 -- Position Sensor/RConn2
  Position Sensor/RConn1 -- Frame/RConn1
  PS-Simulink Converter1/LConn1 -- Position Sensor/RConn3
  Position Sensor/LConn1 -- World Frame/RConn1

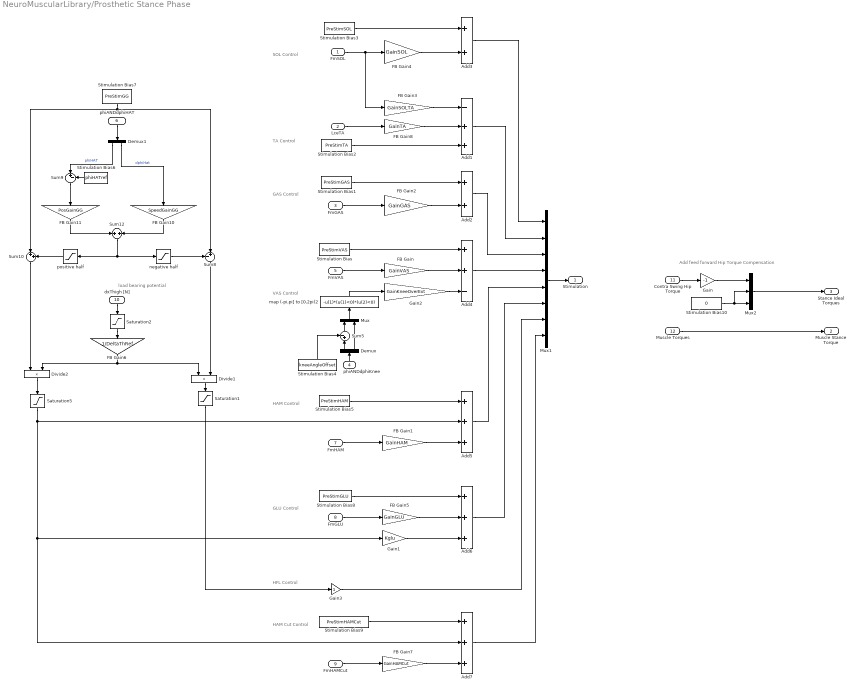
== system NeuroMuscularLibrary/Prosthetic Stance Phase ==
  note: Add feed forward Hip Torque Compensation
  note: load bearing potential
  note: HFL Control
  note: GLU Control
  note: VAS Control
  note: HAM Control
  note: GAS Control
  note: TA Control
  note: SOL Control
  note: HAM Cut Control
  FmSOL : Inport
  LceTA : Inport  Port=2
  FmGAS : Inport  Port=3
  phiANDdphiKnee : Inport  Port=4
  FmVAS : Inport  Port=5
  phiANDdphiHAT : Inport  Port=6
  FmHAM : Inport  Port=7
  FmGLU : Inport  Port=8
  FmHAMCut : Inport  Port=9
  dxThigh [N] : Inport  Port=10
  Contra Swing Hip Torque : Inport  Port=11
  Muscle Torques : Inport  Port=12
  Add1 : Sum  Inputs=-++
  Add2 : Sum
  Add3 : Sum
  Add4 : Sum  Inputs=++-
  Add5 : Sum  Inputs=+++
  Add6 : Sum  Inputs=+++
  Add7 : Sum  Inputs=+++
  Demux : Demux  Outputs=2
  Demux1 : Demux  Outputs=2
  Divide1 : Product
  Divide2 : Product
  FB Gain : Gain  Gain=GainVAS  SaturateOnIntegerOverflow=on  OutDataTypeStr=Inherit: Same as input  ParamDataTypeStr=Inherit: Same as input
  FB Gain1 : Gain  Gain=GainHAM  SaturateOnIntegerOverflow=on  OutDataTypeStr=Inherit: Same as input  ParamDataTypeStr=Inherit: Same as input
  FB Gain10 : Gain  Gain=SpeedGainGG  SaturateOnIntegerOverflow=on  OutDataTypeStr=Inherit: Same as input  ParamDataTypeStr=Inherit: Same as input
  FB Gain11 : Gain  Gain=PosGainGG  SaturateOnIntegerOverflow=on  OutDataTypeStr=Inherit: Same as input  ParamDataTypeStr=Inherit: Same as input
  FB Gain2 : Gain  Gain=GainGAS  SaturateOnIntegerOverflow=on  OutDataTypeStr=Inherit: Same as input  ParamDataTypeStr=Inherit: Same as input
  FB Gain3 : Gain  Gain=GainSOLTA  SaturateOnIntegerOverflow=on  OutDataTypeStr=Inherit: Same as input  ParamDataTypeStr=Inherit: Same as input
  FB Gain4 : Gain  Gain=GainSOL  SaturateOnIntegerOverflow=on  OutDataTypeStr=Inherit: Same as input  ParamDataTypeStr=Inherit: Same as input
  FB Gain5 : Gain  Gain=GainGLU  SaturateOnIntegerOverflow=on  OutDataTypeStr=Inherit: Same as input  ParamDataTypeStr=Inherit: Same as input
  FB Gain6 : Gain  Gain=1/DeltaThRef  SaturateOnIntegerOverflow=on  OutDataTypeStr=Inherit: Same as input  ParamDataTypeStr=Inherit: Same as input
  FB Gain7 : Gain  Gain=GainHAMCut  SaturateOnIntegerOverflow=on  OutDataTypeStr=Inherit: Same as input  ParamDataTypeStr=Inherit: Same as input
  FB Gain8 : Gain  Gain=GainTA  SaturateOnIntegerOverflow=on  OutDataTypeStr=Inherit: Same as input  ParamDataTypeStr=Inherit: Same as input
  Gain : Gain  Gain=-1
  Gain1 : Gain  Gain=Kglu
  Gain2 : Gain  Gain=GainKneeOverExt
  Gain3 : Gain
  Mux : Mux  Inputs=2
  Mux1 : Mux  Inputs=8
  Mux2 : Mux  Inputs=3
  Saturation1 : Saturate  UpperLimit=1  LowerLimit=0  ZeroCross=off
  Saturation2 : Saturate  UpperLimit=inf  LowerLimit=0  ZeroCross=off
  Saturation5 : Saturate  UpperLimit=1  LowerLimit=0  ZeroCross=off
  Stimulation Bias : Constant  Value=PreStimVAS
  Stimulation Bias1 : Constant  Value=PreStimGAS
  Stimulation Bias10 : Constant  Value=0
  Stimulation Bias2 : Constant  Value=PreStimTA
  Stimulation Bias3 : Constant  Value=PreStimSOL
  Stimulation Bias4 : Constant  Value=kneeAngleOffset
  Stimulation Bias5 : Constant  Value=PreStimHAM
  Stimulation Bias6 : Constant  Value=phiHATref
  Stimulation Bias7 : Constant  Value=PreStimGG
  Stimulation Bias8 : Constant  Value=PreStimGLU
  Stimulation Bias9 : Constant  Value=PreStimHAMCut
  Sum10 : Sum  Inputs=|++  SaturateOnIntegerOverflow=on  InputSameDT=on  OutDataTypeStr=Inherit: Same as first input
  Sum12 : Sum  SaturateOnIntegerOverflow=on  InputSameDT=on  OutDataTypeStr=Inherit: Same as first input
  Sum5 : Sum  Inputs=-+|  SaturateOnIntegerOverflow=on  InputSameDT=on  OutDataTypeStr=Inherit: Same as first input
  Sum8 : Sum  Inputs=-+|  SaturateOnIntegerOverflow=on  InputSameDT=on  OutDataTypeStr=Inherit: Same as first input
  Sum9 : Sum  Inputs=|+-  SaturateOnIntegerOverflow=on  InputSameDT=on  OutDataTypeStr=Inherit: Same as first input
  map (-pi,pi] to [0,2pi)2 : Fcn  Expr=-u(1)*(u(1)<0)*(u(2)<0)
  negative half : Saturate  UpperLimit=0  LowerLimit=-inf  ZeroCross=off
  positive half : Saturate  UpperLimit=inf  LowerLimit=0  ZeroCross=off
  Stimulation : Outport
  Muscle Stance Torque : Outport  Port=2
  Stance Ideal Torques : Outport  Port=3
  wires:
  Muscle Torques/1 -> Muscle Stance Torque/1
  Mux2/1 -> Stance Ideal Torques/1
  Stimulation Bias10/1 -> Mux2/2, Mux2/3
  Contra Swing Hip Torque/1 -> Gain/1
  Gain/1 -> Mux2/1
  Add4/1 -> Mux1/4
  Mux1/1 -> Stimulation/1
  Gain1/1 -> Add6/3
  FB Gain5/1 -> Add6/2
  Stimulation Bias8/1 -> Add6/1
  Add6/1 -> Mux1/6
  Add5/1 -> Mux1/5
  FB Gain1/1 -> Add5/3
  Stimulation Bias5/1 -> Add5/1
  Stimulation Bias/1 -> Add4/1
  Stimulation Bias1/1 -> Add2/1
  Add2/1 -> Mux1/3
  Stimulation Bias2/1 -> Add1/3
  Stimulation Bias3/1 -> Add3/1
  FmGLU/1 -> FB Gain5/1
  FmHAM/1 -> FB Gain1/1
  map (-pi,pi] to [0,2pi)2/1 -> Gain2/1
  Sum8/1 -> Divide1/2
  Sum10/1 -> Divide2/1
  Sum9/1 -> FB Gain11/1
  FB Gain6/1 -> Divide1/1, Divide2/2
  Divide2/1 -> Saturation5/1
  Divide1/1 -> Saturation1/1
  Saturation1/1 -> Gain3/1
  dxThigh [N]/1 -> Saturation2/1
  Saturation2/1 -> FB Gain6/1
  Gain3/1 -> Mux1/7
  Gain2/1 -> Add4/3
  negative half/1 -> Sum8/1
  Sum12/1 -> negative half/1, positive half/1
  positive half/1 -> Sum10/2
  Demux1/2 -> FB Gain10/1  "dphiHat"
  Demux1/1 -> Sum9/1  "phiHAT"
  phiANDdphiHAT/1 -> Demux1/1
  FB Gain10/1 -> Sum12/2
  FB Gain11/1 -> Sum12/1
  Stimulation Bias7/1 -> Sum8/2, Sum10/1
  Stimulation Bias6/1 -> Sum9/2
  Stimulation Bias4/1 -> Sum5/1
  Demux/2 -> Mux/2
  Demux/1 -> Sum5/2
  phiANDdphiKnee/1 -> Demux/1
  Sum5/1 -> Mux/1
  Mux/1 -> map (-pi,pi] to [0,2pi)2/1
  FmVAS/1 -> FB Gain/1
  FB Gain/1 -> Add4/2
  FB Gain2/1 -> Add2/2
  FmGAS/1 -> FB Gain2/1
  LceTA/1 -> FB Gain8/1
  FB Gain8/1 -> Add1/2
  Add1/1 -> Mux1/2
  FB Gain3/1 -> Add1/1
  FmSOL/1 -> FB Gain3/1, FB Gain4/1
  FB Gain4/1 -> Add3/2
  Add3/1 -> Mux1/1
  Add7/1 -> Mux1/8
  FB Gain7/1 -> Add7/3
  Stimulation Bias9/1 -> Add7/1
  FmHAMCut/1 -> FB Gain7/1
  Saturation5/1 -> Add5/2, Add7/2, Gain1/1

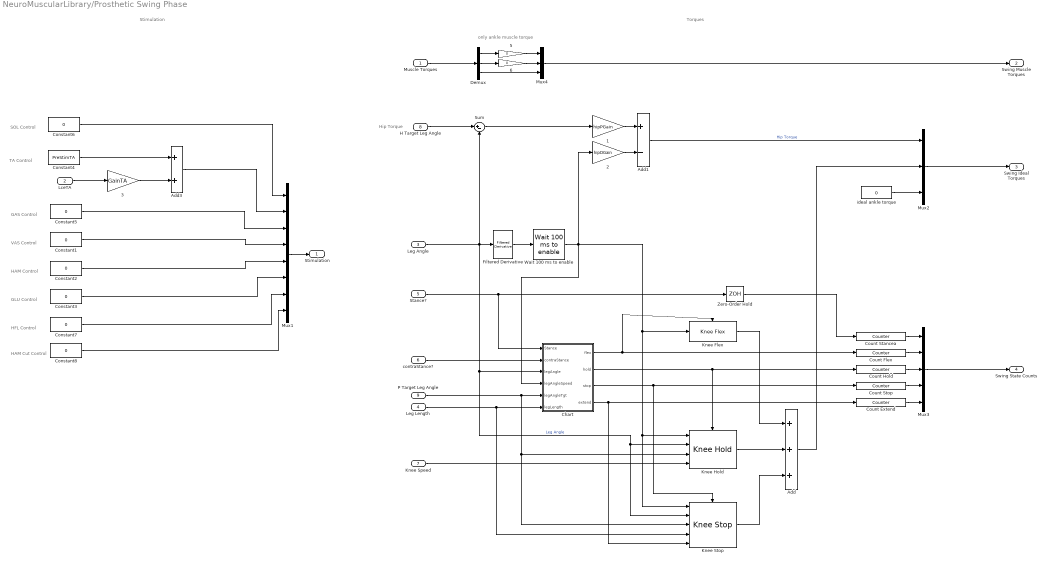
== system NeuroMuscularLibrary/Prosthetic Swing Phase ==
  note: Hip Torque
  note: only ankle muscle torque
  note: HAM Cut
      | Control
  note: Torques
  note: HFL Control
  note: GLU Control
  note: HAM Control
  note: VAS Control
  note: TA Control
  note: GAS Control
  note: SOL Control
  note: Stimulation
  Muscle Torques : Inport
  LceTA : Inport  Port=2
  Leg Angle : Inport  Port=3
  Leg Length : Inport  Port=4
  Stance? : Inport  Port=5
  contraStance? : Inport  Port=6
  Knee Speed : Inport  Port=7
  H Target Leg Angle : Inport  Port=8
  P Target Leg Angle : Inport  Port=9
  " 1" : Gain  Gain=hipPGain
  " 2" : Gain  Gain=hipDGain
  " 3" : Gain  Gain=GainTA
  " 5" : Gain  Gain=0
  " 6" : Gain  Gain=0
  Add : Sum  Inputs=+++
  Add1 : Sum  Inputs=+-
  Add3 : Sum
  Chart : Stateflow chart  TreatAsAtomicUnit=on
  Constant{1..3,5..8} (7 alike) : Constant  Value=0
  Constant4 : Constant  Value=PreStimTA
  Count Extend : dspswit3/Counter  Direction=Up  CountEvent=Rising edge  CounterSize=16 bits  MaxCount=255  InitialCount=0  Output=Count  HitValue=32  ResetInput=off  SamplesPerFrame=1  Ts=1  CntDtype=double  HitDtype=Logical
  Count Flex : dspswit3/Counter  Direction=Up  CountEvent=Rising edge  CounterSize=16 bits  MaxCount=255  InitialCount=0  Output=Count  HitValue=32  ResetInput=off  SamplesPerFrame=1  Ts=1  CntDtype=double  HitDtype=Logical
  Count Hold : dspswit3/Counter  Direction=Up  CountEvent=Rising edge  CounterSize=16 bits  MaxCount=255  InitialCount=0  Output=Count  HitValue=32  ResetInput=off  SamplesPerFrame=1  Ts=1  CntDtype=double  HitDtype=Logical
  Count Stancea : dspswit3/Counter  Direction=Up  CountEvent=Rising edge  CounterSize=16 bits  MaxCount=255  InitialCount=0  Output=Count  HitValue=32  ResetInput=off  SamplesPerFrame=1  Ts=1  CntDtype=double  HitDtype=Logical
  Count Stop : dspswit3/Counter  Direction=Up  CountEvent=Rising edge  CounterSize=16 bits  MaxCount=255  InitialCount=0  Output=Count  HitValue=32  ResetInput=off  SamplesPerFrame=1  Ts=1  CntDtype=double  HitDtype=Logical
  Demux : Demux  Outputs=3
  Filtered Derivative : NeuroMuscularLibrary/Swing Phase/Filtered Derivative
  Knee Flex : NeuroMuscularLibrary/Swing Phase/Knee Flex
  Knee Hold : NeuroMuscularLibrary/Swing Phase/Knee Hold
  Knee Stop : NeuroMuscularLibrary/Swing Phase/Knee Stop
  Mux1 : Mux  Inputs=8
  Mux2 : Mux  Inputs=3
  Mux3 : Mux  Inputs=5
  Mux4 : Mux  Inputs=3
  Sum : Sum  Inputs=|+-
  Wait 100 ms to enable : NeuroMuscularLibrary/Swing Phase/Wait 100 ms to enable
  Zero-Order Hold : ZeroOrderHold  SampleTime=.01
  ideal ankle torque : Constant  Value=0
  Stimulation : Outport
  Swing Muscle Torques : Outport  Port=2
  Swing Ideal Torques : Outport  Port=3
  Swing State Counts : Outport  Port=4
  wires:
  P Target Leg Angle/1 -> Chart/5(legAngleTgt), Knee Hold/3, Knee Stop/3
  Mux2/1 -> Swing Ideal Torques/1
  ideal ankle torque/1 -> Mux2/3
  Zero-Order Hold/1 -> Count Stancea/1
  Count Stancea/1 -> Mux3/1
  Mux3/1 -> Swing State Counts/1
  Count Flex/1 -> Mux3/2
  Count Hold/1 -> Mux3/3
  Count Stop/1 -> Mux3/4
  Count Extend/1 -> Mux3/5
  Add1/1 -> Mux2/1  "Hip Torque"
  Leg Length/1 -> Knee Stop/4, Chart/6(legLength)
  contraStance?/1 -> Chart/2(contraStance)
  Stance?/1 -> Chart/1(Stance), Zero-Order Hold/1
  Chart/4(extend) -> Knee Stop/5, Count Extend/1
  Chart/3(stop) -> Knee Stop/Enable, Count Stop/1
  Chart/2(hold) -> Knee Hold/Enable, Count Hold/1
  Chart/1(flex) -> Count Flex/1, Knee Flex/Enable
  Add/1 -> Mux2/2
  Knee Stop/1 -> Add/3
  Knee Flex/1 -> Add/1
  Knee Hold/1 -> Add/2
  Knee Speed/1 -> Knee Hold/4
  Leg Angle/1 -> Sum/2, Knee Hold/2, Knee Stop/2, Chart/3(legAngle), Filtered Derivative/1  "Leg Angle"
  Sum/1 -> " 1"/1
  " 1"/1 -> Add1/1
  " 2"/1 -> Add1/2
  H Target Leg Angle/1 -> Sum/1
  Filtered Derivative/1 -> Wait 100 ms to enable/1
  Wait 100 ms to enable/1 -> " 2"/1, Knee Flex/1, Knee Stop/1, Knee Hold/1, Chart/4(legAngleSpeed)
  Demux/3 -> Mux4/3
  " 6"/1 -> Mux4/2
  " 5"/1 -> Mux4/1
  Demux/2 -> " 6"/1
  Demux/1 -> " 5"/1
  Muscle Torques/1 -> Demux/1
  Mux4/1 -> Swing Muscle Torques/1
  Constant8/1 -> Mux1/8
  Mux1/1 -> Stimulation/1
  Constant7/1 -> Mux1/7
  Constant3/1 -> Mux1/6
  Constant2/1 -> Mux1/5
  Constant1/1 -> Mux1/4
  Constant5/1 -> Mux1/3
  Constant6/1 -> Mux1/1
  Add3/1 -> Mux1/2
  LceTA/1 -> " 3"/1
  " 3"/1 -> Add3/2
  Constant4/1 -> Add3/1

== system NeuroMuscularLibrary/SOL Link ==
  note: Soleus Attachment
  Ankle Angle [rad] : Inport
  Constant : Constant  Value=lslackSOL+loptSOL
  Constant2 : Constant  Value=phirefSOL
  Constant3 : Constant  Value=phimaxSOL
  Demux : Demux  Outputs=2
  Gain2 : Gain  Gain=rSOL
  Gain4 : Gain  Gain=rhoSOL
  Mux : Mux  Inputs=2
  Sum2 : Sum  Inputs=|+-
  Sum3 : Sum  Inputs=-+|
  Sum4 : Sum  Inputs=+-
  Sum5 : Sum  Inputs=|++
  length change term : Trigonometry
  offset correction term : Trigonometry
  variable lever term : Trigonometry  Operator=cos
  lmtc [m] : Outport
  lever [m] : Outport  Port=2
  wires:
  Ankle Angle [rad]/1 -> Sum3/2
  Sum3/1 -> variable lever term/1, length change term/1
  Constant3/1 -> Sum3/1, Sum2/2
  Sum2/1 -> offset correction term/1
  Constant2/1 -> Sum2/1
  length change term/1 -> Sum4/2
  offset correction term/1 -> Sum4/1
  Sum4/1 -> Mux/1
  Constant/1 -> Sum5/1
  Sum5/1 -> lmtc [m]/1
  Gain4/1 -> Sum5/2
  variable lever term/1 -> Mux/2
  Mux/1 -> Gain2/1
  Gain2/1 -> Demux/1
  Demux/1 -> Gain4/1
  Demux/2 -> lever [m]/1

== system NeuroMuscularLibrary/Sensor Sheet ==
  note: Inner Segment Pressure Sheet
  Gain3 : Gain  Gain=k_pressure
  Gain4 : Gain  Gain=1/v_max_pressure
  Mux1 : Mux  Inputs=2
  PS-Simulink Converter : nesl_utility/PS-Simulink Converter  PhysicalDomain=network_engine_domain  SubClassName=ps_output  LeftPortType=input  RightPortType=output  PseudoPeriodic=off  Frequencies=[]  Unit=1  AffineConversion=off
  PS-Simulink Converter1 : nesl_utility/PS-Simulink Converter  PhysicalDomain=network_engine_domain  SubClassName=ps_output  LeftPortType=input  RightPortType=output  PseudoPeriodic=off  Frequencies=[]  Unit=1  AffineConversion=off
  Pressure Sheet Reaction Force : Fcn  Expr=-u(1) * (1+sgn(u(1))*u(2))
  Prismatic Joint : sm_lib/Joints/Prismatic Joint  SenseConstraintForce=off  SenseConstraintForceX=off  SenseConstraintForceY=off  SenseConstraintForceZ=off  SenseConstraintTorque=off  SenseConstraintTorqueX=off  SenseConstraintTorqueY=off  SenseConstraintTorqueZ=off  SenseTotalForce=off  SenseTotalForceX=off  SenseTotalForceY=off  SenseTotalForceZ=off  SenseTotalTorque=off  SenseTotalTorqueX=off  SenseTotalTorqueY=off  SenseTotalTorqueZ=off  CompositeWrenchDir=FollowerOnBase  CompositeWrenchFrame=BaseFrame  EquilibriumPosition=0  EquilibriumPositionUnits=m  SpringStiffness=0  SpringStiffnessUnits=N/m  DampingCoefficient=0  DampingCoefficientUnits=N/(m/s)  TorqueActuationMode=InputTorque  MotionActuationMode=ComputedMotion  SensePosition=on  SenseVelocity=on  SenseAcceleration=off  SenseTorqueForce=off  PositionTargetValue=0  PositionTargetValueUnits=m  PositionTargetSpecify=on  PositionTargetPriority=High  VelocityTargetValue=0  VelocityTargetValueUnits=m/s  VelocityTargetSpecify=on  VelocityTargetPriority=High  BlockFunction=simmechanics.library.joints.prismatic_joint
  Simulink-PS Converter : nesl_utility/Simulink-PS Converter  PhysicalDomain=network_engine_domain  SubClassName=ps_input  LeftPortType=input  RightPortType=output  PseudoPeriodic=off  Frequencies=[]  NoiseDistribution=none  NoiseParameters=[]  Unit=1  AffineConversion=off  InputFiltering=off  SimscapeFilterOrder=1  InputFilterTimeConstant=0.001  UdotUserProvided=1
  Y-up TO Z-up : sm_lib/Frames and Transforms/Rigid Transform  TranslationMethod=None  TranslationLengthUnit=m  TranslationStandardAxis=+Z  TranslationStandardOffset=0  TranslationCartesianOffset=[0 0 0]  TranslationROffset=0  TranslationROffsetUnits=m  TranslationZOffset=0  TranslationZOffsetUnits=m  TranslationThetaOffset=0  TranslationThetaOffsetUnits=deg  RotationMethod=AlignedAxes  RotationAngleUnits=deg  RotationStandardAxis=+Z  RotationAngle=0  RotationArbitraryAxis=[0 0 1]  FollAlignAxisA=+X  BaseAlignAxisA=+X  FollAlignAxisB=+Z  BaseAlignAxisB=+Y  RotationMatrix=[1 0 0; 0 1 0; 0 0 1]  BlockFunction=simmechanics.library.frames_transforms.rigid_transform
  Z-up TO Y-up : sm_lib/Frames and Transforms/Rigid Transform  TranslationMethod=None  TranslationLengthUnit=m  TranslationStandardAxis=+Z  TranslationStandardOffset=0  TranslationCartesianOffset=[0 0 0]  TranslationROffset=0  TranslationROffsetUnits=m  TranslationZOffset=0  TranslationZOffsetUnits=m  TranslationThetaOffset=0  TranslationThetaOffsetUnits=deg  RotationMethod=AlignedAxes  RotationAngleUnits=deg  RotationStandardAxis=+Z  RotationAngle=0  RotationArbitraryAxis=[0 0 1]  FollAlignAxisA=+X  BaseAlignAxisA=+X  FollAlignAxisB=+Y  BaseAlignAxisB=+Z  RotationMatrix=[1 0 0; 0 1 0; 0 0 1]  BlockFunction=simmechanics.library.frames_transforms.rigid_transform
  Thigh : PMIOPort  Port=1  Side=Left
  Hip Joint : PMIOPort  Port=2  Side=Right
  dx : Outport
  wires:
  PS-Simulink Converter/1 -> Gain3/1, dx/1  "position"
  PS-Simulink Converter1/1 -> Gain4/1  "velocity"
  Mux1/1 -> Pressure Sheet Reaction Force/1
  Gain3/1 -> Mux1/1
  Gain4/1 -> Mux1/2
  Pressure Sheet Reaction Force/1 -> Simulink-PS Converter/1
  connections:
  Prismatic Joint/LConn1 -- Y-up TO Z-up/RConn1
  Prismatic Joint/RConn1 -- Z-up TO Y-up/LConn1
  Prismatic Joint/LConn2 -- Simulink-PS Converter/RConn1
  Prismatic Joint/RConn2 -- PS-Simulink Converter/LConn1
  Prismatic Joint/RConn3 -- PS-Simulink Converter1/LConn1
  Y-up TO Z-up/LConn1 -- Thigh/RConn1
  Hip Joint/RConn1 -- Z-up TO Y-up/RConn1

== system NeuroMuscularLibrary/Shank ==
  Ankle to Center : sm_lib/Frames and Transforms/Rigid Transform  TranslationMethod=Cartesian  TranslationLengthUnit=m  TranslationStandardAxis=+Z  TranslationStandardOffset=0  TranslationCartesianOffset=[0 shankAnkleToCenterDist 0]  TranslationROffset=0  TranslationROffsetUnits=m  TranslationZOffset=0  TranslationZOffsetUnits=m  TranslationThetaOffset=0  TranslationThetaOffsetUnits=deg  RotationMethod=AlignedAxes  RotationAngleUnits=deg  RotationStandardAxis=+Z  RotationAngle=0  RotationArbitraryAxis=[0 0 1]  FollAlignAxisA=+Z  BaseAlignAxisA=+Y  FollAlignAxisB=+X  BaseAlignAxisB=+X  RotationMatrix=[1 0 0; 0 1 0; 0 0 1]  BlockFunction=simmechanics.library.frames_transforms.rigid_transform
  Ankle to Knee : sm_lib/Frames and Transforms/Rigid Transform  TranslationMethod=Cartesian  TranslationLengthUnit=m  TranslationStandardAxis=+Z  TranslationStandardOffset=0  TranslationCartesianOffset=[0 shankAnkleToKneeDist 0]  TranslationROffset=0  TranslationROffsetUnits=m  TranslationZOffset=0  TranslationZOffsetUnits=m  TranslationThetaOffset=0  TranslationThetaOffsetUnits=deg  RotationMethod=None  RotationAngleUnits=deg  RotationStandardAxis=+Z  RotationAngle=0  RotationArbitraryAxis=[0 0 1]  FollAlignAxisA=+Z  BaseAlignAxisA=+Z  FollAlignAxisB=+X  BaseAlignAxisB=-X  RotationMatrix=[1 0 0; 0 1 0; 0 0 1]  BlockFunction=simmechanics.library.frames_transforms.rigid_transform
  Shank Center to CG : sm_lib/Frames and Transforms/Rigid Transform  TranslationMethod=Cartesian  TranslationLengthUnit=m  TranslationStandardAxis=+Z  TranslationStandardOffset=0  TranslationCartesianOffset=[0 0 shankCenterToCGDist]  TranslationROffset=0  TranslationROffsetUnits=m  TranslationZOffset=0  TranslationZOffsetUnits=m  TranslationThetaOffset=0  TranslationThetaOffsetUnits=deg  RotationMethod=None  RotationAngleUnits=deg  RotationStandardAxis=+Z  RotationAngle=0  RotationArbitraryAxis=[0 0 1]  FollAlignAxisA=+X  BaseAlignAxisA=+Y  FollAlignAxisB=+Y  BaseAlignAxisB=+Z  RotationMatrix=[1 0 0; 0 1 0; 0 0 1]  BlockFunction=simmechanics.library.frames_transforms.rigid_transform
  Shank Solid : sm_lib/Body Elements/Solid  InertiaType=Custom  Mass=shankMass  MassUnits=kg  CenterOfMass=[0 0 shankCenterToCGDist]  CenterOfMassUnits=m  MomentsOfInertia=[shankInertia 0 0]  MomentsOfInertiaUnits=kg*m^2  ProductsOfInertia=[0 0 0]  ProductsOfInertiaUnits=kg*m^2  DensityBased=on  Density=1000  DensityUnits=kg/(m^3)  GraphicType=FromGeometry  MarkerShape=Sphere  MarkerSize=10  MarkerSizeUnits=m  GraphicVisPropType=SimpleVisualProperties  GraphicDiffuseColor=[0.5 0.5 0.5]  GraphicSpecularColor=[0.5 0.5 0.5 1.0]  GraphicAmbientColor=[0.15 0.15 0.15 1.0]  GraphicEmissiveColor=[0.0 0.0 0.0 1.0]  GraphicShininess=75  GraphicOpacity=1.0  GeometryShape=Cylinder  RectangleSize=[1 1]  RectangleSizeUnits=m  BrickDimensions=[1.05 .1]  BrickDimensionUnits=m  CylinderRadius=.04  CylinderRadiusUnits=m  CylinderLength=shankLength  CylinderLengthUnits=m  SphereRadius=1  SphereRadiusUnits=m  EllipsoidRadii=[1 1 1]  EllipsoidRadiiUnits=m  ExtrusionCrossSection=[1 1; -1 1; -1 -1; 1 -1]  ExtrusionCrossSectionUnits=m  ExtrusionLength=1  ExtrusionLengthUnits=m  PolygonNumSides=3  PolygonOuterRadius=1  PolygonOuterRadiusUnits=m  ExtGeomFileType=STL  ExtGeomFileUnits=m  RevolutionCrossSection=[1 1; 1 -1; 2 -1; 2 1]  RevolutionCrossSectionUnits=m  RevolutionExtent=Full  RevolutionAngle=180  RevolutionAngleUnits=deg  BlockFunction=simmechanics.library.body_elements.solid
  Ankle : PMIOPort  Port=1  Side=Left
  Knee : PMIOPort  Port=2  Side=Right
  CG : PMIOPort  Port=3  Side=Left
  connections:
  Ankle to Knee/LConn1 -- Ankle/RConn1 -- Ankle to Center/LConn1
  Shank Solid/RConn1 -- Ankle to Center/RConn1 -- Shank Center to CG/LConn1
  Ankle to Knee/RConn1 -- Knee/RConn1
  CG/RConn1 -- Shank Center to CG/RConn1
